simulink model "modelArduino"  (R2015a)
settings: Solver=ode3  StartTime=0.0  StopTime=10.0  FixedStep=1/200  RelTol=1e-3
values from neighbouring files (symbols this model uses):
  K = dlqr(plant.a, plant.b,diag([0,0,0,1,0.1,0,0]), 1)    [Untitled2.m]
undefined symbols (not defined in the file or in its folder): Discrete, plant, R, Time
libraries: PoliArd x8, ctrlSharedLib x1
settings Model: ExtModeTrigDuration=2  Creator=User  LastModifiedBy=user
settings OptimizationCC: OptimizeModelRefInitCode=on  LifeSpan=1
settings DebuggingCC: UnderspecifiedInitializationDetection=Classic  MergeDetectMultiDrivingBlocksExec=none
settings HardwareCC: ProdLargestAtomicInteger=Long  ProdLargestAtomicFloat=Double  ProdEndianess=LittleEndian  ProdHWDeviceType=ARM Compatible->ARM Cortex
settings RTWCC: SystemTargetFile=realtime.tlc  GenerateMakefile=off  TemplateMakefile=realtime.tmf  Description=Run on Target Hardware  RTWVerbose=off
settings ERTTargetCC: CombineOutputUpdateFcns=off  ExtModeTransport=3  ExtModeMexFile=ext_serial_win32_comm_rtt  ExtModeMexArgs=0 1 9600  ERTSrcFileBannerTemplate=realtime_code_template.cgt  ERTHdrFileBannerTemplate=realtime_code_template.cgt  ERTDataSrcFileTemplate=realtime_code_template.cgt  ERTDataHdrFileTemplate=realtime_code_template.cgt  ERTCustomFileTemplate=realtime_file_process.tlc

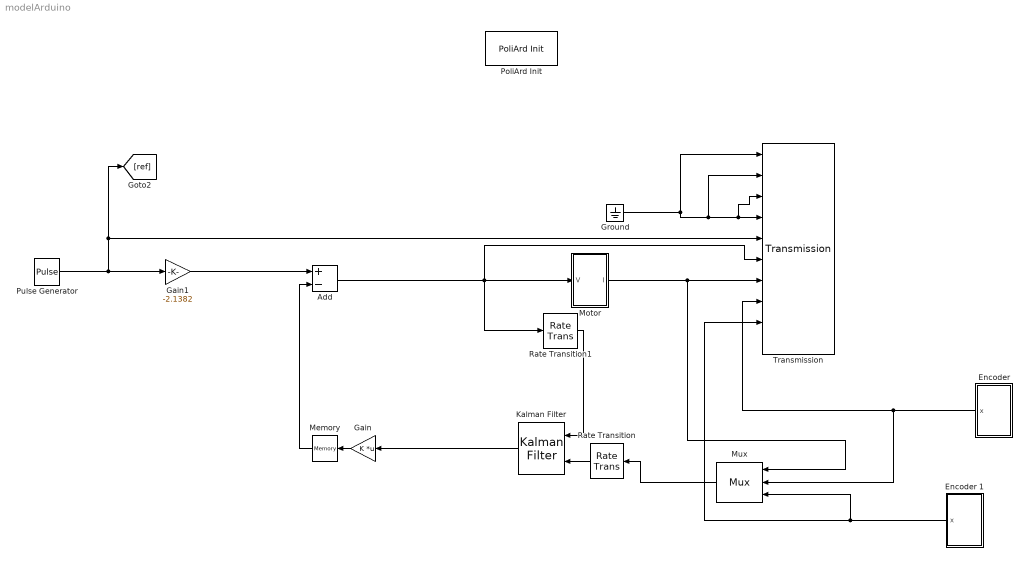
== system modelArduino ==
  Add : Sum  Inputs=+-
  "Encoder " : Subsystem
  Encoder 1 : Subsystem
  Gain : Gain  Gain=K  Multiplication=Matrix(K*u)
  Gain1 : Gain  Gain=-2.1382
  Ground : Ground
  Kalman Filter : ctrlSharedLib/Kalman Filter  TimeDomain=Discrete-Time  UseCurrentEstimator=on  ModelSource=Individual A, B, C, D matrices  ModelSourceVariable=ss(0.95,1,1,0,1)  A=plant.a  B=plant.b  C=plant.c  D=plant.d  NumberOfStates=1  NumberOfInputs=1  NumberOfOutputs=1  InitialEstimateSource=Dialog  X0=0  P0=10  UseK=off  UseGH=off  NumberOfProcessNoiseInputs=1  G=1  TimeInvariantG=on  H=0  TimeInvariantH=on  Q=Q  TimeInvariantQ=on  R=R  TimeInvariantR=on  N=0  TimeInvariantN=on  AddInputPort=on  AddEnablePort=off  OutputEstimatedY=off  OutputP=off  Ts=1/200
  Memory : Memory
  Motor : Subsystem
  Mux : Mux  Inputs=3
  PoliArd Init : PoliArd/PoliArd Init
  Pulse Generator : DiscretePulseGenerator  PulseType=Time based  Period=10  PulseWidth=50  PhaseDelay=5
  Rate Transition : RateTransition  OutPortSampleTime=1/200
  Rate Transition1 : RateTransition  OutPortSampleTime=1/200
  Transmission : PoliArd/Transmission  sample_freq=200  sig_to_send=6
  wires:
  Ground/1 -> Transmission/2, Transmission/3, Transmission/4, Transmission/1
  Motor/1(I) -> Transmission/7, Mux/1
  Kalman Filter/1 -> Gain/1
  Gain1/1 -> Add/1
  Pulse Generator/1 -> Gain1/1, [ref], Transmission/5
  "Encoder "/1(x) -> Mux/2, Transmission/8
  Gain/1 -> Memory/1
  Add/1 -> Rate Transition1/1, Transmission/6, Motor/1(V)
  Rate Transition1/1 -> Kalman Filter/1
  Memory/1 -> Add/2
  Encoder 1/1(x) -> Mux/3, Transmission/9
  Mux/1 -> Rate Transition/1
  Rate Transition/1 -> Kalman Filter/2

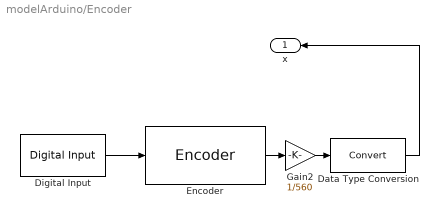
== system modelArduino/Encoder  ==
  Data Type Conversion : DataTypeConversion
  Digital Input : PoliArd/Digital Input  DI_pin=2  DIsample=1/200
  Encoder : PoliArd/Encoder  EncoderID=1  dt_enc=1/200
  Gain2 : Gain  Gain=1/560
  x : Outport
  wires:
  Digital Input/1 -> Encoder/1
  Encoder/1 -> Gain2/1
  Gain2/1 -> Data Type Conversion/1
  Data Type Conversion/1 -> x/1

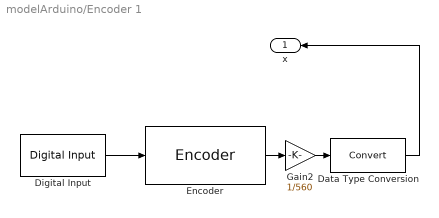
== system modelArduino/Encoder 1 ==
  Data Type Conversion : DataTypeConversion
  Digital Input : PoliArd/Digital Input  DI_pin=2  DIsample=1/200
  Encoder : PoliArd/Encoder  EncoderID=4  dt_enc=1/200
  Gain2 : Gain  Gain=1/560
  x : Outport
  wires:
  Digital Input/1 -> Encoder/1
  Encoder/1 -> Gain2/1
  Gain2/1 -> Data Type Conversion/1
  Data Type Conversion/1 -> x/1

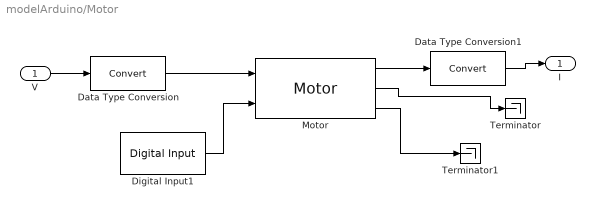
== system modelArduino/Motor ==
  V : Inport
  Data Type Conversion : DataTypeConversion
  Data Type Conversion1 : DataTypeConversion
  Digital Input1 : PoliArd/Digital Input  DI_pin=3  DIsample=1/200
  Motor : PoliArd/Motor  MotorID=2  DC_bus_mask=12  dt_mot=1/200
  Terminator : Terminator
  Terminator1 : Terminator
  I : Outport
  wires:
  Data Type Conversion/1 -> Motor/1
  Digital Input1/1 -> Motor/2
  V/1 -> Data Type Conversion/1
  Motor/3 -> Terminator1/1
  Motor/2 -> Terminator/1
  Motor/1 -> Data Type Conversion1/1
  Data Type Conversion1/1 -> I/1
